simulink model "sprung"  (Simulink 8.2)
settings: Solver=ode4  StartTime=0.0  StopTime=10.0  FixedStep=0.01  RelTol=1e-3
model workspace: external: MAT-File sprung_ws.mat (data not in the file)
values from neighbouring files (symbols this model uses):
  D = outputs.fcn.D    [sprung_plot.m]    (also in sprung_ws.mat = 132.25)
  N = [1 5.5271 10.1848 7.8258 0]    [sprung_ws.mat]
  Tbase = outputs.mdl.Tbase    [sprung_plot.m]    (also in sprung_ws.mat = 5)
  Z = [-625.154 -1315.1998 -1030.7301 0.2116]    [sprung_ws.mat]
settings Model: Creator=abb344  LastModifiedBy=Kira
settings DataIOCC: MaxDataPoints=Smp  SignalLoggingSaveFormat=Dataset  TimeSaveName=t  OutputSaveName=u_y_dy
settings DebuggingCC: InheritedTsInSrcMsg=none  FcnCallInpInsideContextMsg=EnableAllAsError
settings GRTTargetCC: CombineOutputUpdateFcns=on  GRTInterface=off

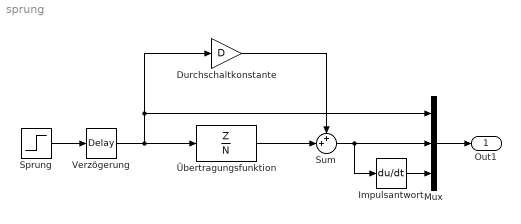
== system sprung ==
  Durchschaltkonstante : Gain  Gain=D
  Impulsantwort : Derivative
  Mux : Mux  Inputs=3
  Sprung : Step  Time=-1
  Sum : Sum  Inputs=++|
  Verzögerung : TransportDelay  DelayTime=Tbase  BufferSize=10000  FixedBuffer=on
  Übertragungsfunktion : TransferFcn  Numerator=Z  Denominator=N
  Out1 : Outport
  wires:
  Durchschaltkonstante/1 -> Sum/1
  Übertragungsfunktion/1 -> Sum/2
  Sprung/1 -> Verzögerung/1
  Mux/1 -> Out1/1
  Sum/1 -> Impulsantwort/1, Mux/2
  Impulsantwort/1 -> Mux/3
  Verzögerung/1 -> Mux/1, Durchschaltkonstante/1, Übertragungsfunktion/1
